simulink model "flyWheel"  (R2018b)
settings: Solver=ode45  StartTime=0.0  StopTime=59  RelTol=1e-3
libraries: simulink x3
settings Model: Creator=ROG  LastModifiedBy=ROG

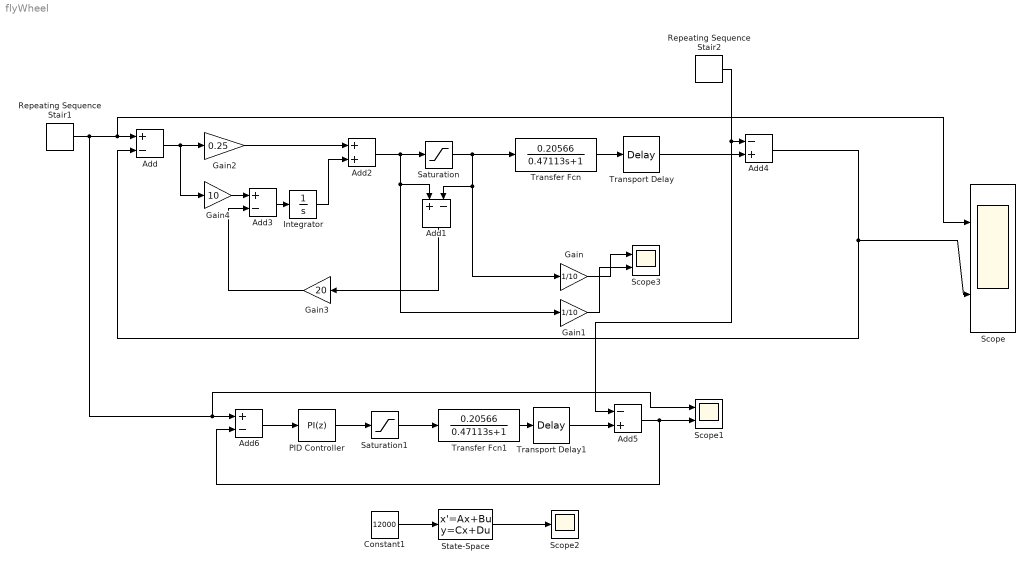
== system flyWheel ==
  Add{,1,3,6} (4 alike) : Sum  Inputs=+-
  Add2 : Sum
  Add4 : Sum  Inputs=-+
  Add5 : Sum  Inputs=-+
  Constant1 : Constant  Value=12000
  Gain : Gain  Gain=1/10
  Gain1 : Gain  Gain=1/10
  Gain2 : Gain  Gain=0.25
  Gain3 : Gain  Gain=20
  Gain4 : Gain  Gain=10
  Integrator : Integrator
  PID Controller : simulink/Continuous/PID Controller  Controller=PI  Form=Parallel  TimeDomain=Discrete-time  SampleTime=0.005  IntegratorMethod=Forward Euler  FilterMethod=Forward Euler  ControllerParametersSource=internal  P=0.25  I=10  D=0  UseFilter=on  N=100  TunerSelectOption=Transfer Function Based (PID Tuner App)  InitialConditionSource=internal  InitialConditionForIntegrator=0  InitialConditionForFilter=0  DifferentiatorICPrevScaledInput=0  ExternalReset=none  TrackingMode=off  Kt=1  LimitOutput=off  UpperSaturationLimit=inf  LowerSaturationLimit=-inf  LinearizeAsGain=on  AntiWindupMode=none  Kb=1  POutMin=[]  POutMax=[]  IOutMin=[]  IOutMax=[]  DOutMin=[]  DOutMax=[]  NOutMin=[]  NOutMax=[]  SumOutMin=[]  SumOutMax=[]  SaturationOutMin=[]  SaturationOutMax=[]  PParamMin=[]  PParamMax=[]  IParamMin=[]  IParamMax=[]  DParamMin=[]  DParamMax=[]  NParamMin=[]  NParamMax=[]  KbParamMin=[]  KbParamMax=[]  KtParamMin=[]  KtParamMax=[]  KbOutMin=[]  KbOutMax=[]  KtOutMin=[]  KtOutMax=[]  IntegratorOutMin=[]  IntegratorOutMax=[]  FilterOutMin=[]  FilterOutMax=[]  SumI1OutMin=[]  SumI1OutMax=[]  SumI2OutMin=[]  SumI2OutMax=[]  SumI3OutMin=[]  SumI3OutMax=[]  SumI4OutMin=[]  SumI4OutMax=[]  SumDOutMin=[]  SumDOutMax=[]  DifferentiatorOutMin=[]  DifferentiatorOutMax=[]  FilterDiffOutCoefMin=[]  FilterDiffOutCoefMax=[]  ReciprocalOutMin=[]  ReciprocalOutMax=[]  SumDenOutMin=[]  SumDenOutMax=[]  SumNumOutMin=[]  SumNumOutMax=[]  DivideOutMin=[]  DivideOutMax=[]  IntegratorContinuousStateAttributes=''  IntegratorStateMustResolveToSignalObject=off  IntegratorRTWStateStorageClass=Auto  FilterContinuousStateAttributes=''  FilterStateMustResolveToSignalObject=off  FilterRTWStateStorageClass=Auto  ParallelPVariant=InternalParameters  IdealPVariant=Disabled  IVariant=InternalParameters  DVariant=Disabled  IntegratorVariant=Discrete  SatVariant=Disabled  AWVariant=Passthrough  PCopyVariant=Disabled  TRVariant=Disabled  FdbkBlocksVariant=Forward  IdealPFdbkVariant=Disabled  SatFdbkVariant=Disabled  DerivativeFilterVariant=Disabled  NVariant=Disabled  NCopyVariant=Disabled_SignalSpec  FilterICVariant=Disabled  IntegratorICVariant=InternalICs  ExternalResetVariant=Disabled  TRSumVariant=Passthrough  SumFdbkVariant=Disabled  SumVariant=Sum_PI
  Repeating Sequence Stair1 : simulink/Sources/Repeating Sequence Stair  OutValues=[1800 800 2500 1800 1800].'  tsamp=10  OutMin=[]  OutMax=[]  OutDataTypeStr=double  OutputDataTypeScalingMode=double  OutDataType=fixdt(0,8)  ConRadixGroup=Best Precision: Vector-wise  OutScaling=2^-12
  Repeating Sequence Stair2 : simulink/Sources/Repeating Sequence Stair  OutValues=[0 0 0 0 600 600]  tsamp=10  OutMin=[]  OutMax=[]  OutDataTypeStr=double  OutputDataTypeScalingMode=double  OutDataType=fixdt(0,8)  ConRadixGroup=Best Precision: Vector-wise  OutScaling=2^-12
  Saturation : Saturate  UpperLimit=12000  LowerLimit=-12000
  Saturation1 : Saturate  UpperLimit=12000  LowerLimit=-12000
  Scope : Scope  NumInputPorts=2
  Scope1 : Scope  NumInputPorts=2
  Scope2 : Scope
  Scope3 : Scope  NumInputPorts=2
  State-Space : StateSpace  A=-2.1226  C=0.4365  D=0  InitialCondition=0
  Transfer Fcn : TransferFcn  Numerator=[0.20566]  Denominator=[0.47113 1]
  Transfer Fcn1 : TransferFcn  Numerator=[0.20566]  Denominator=[0.47113 1]
  Transport Delay : TransportDelay  DelayTime=0.03368
  Transport Delay1 : TransportDelay  DelayTime=0.03368
  wires:
  Transfer Fcn/1 -> Transport Delay/1
  Saturation/1 -> Gain/1, Add1/2, Transfer Fcn/1
  Add2/1 -> Gain1/1, Add1/1, Saturation/1
  Add1/1 -> Gain3/1
  Integrator/1 -> Add2/2
  Add3/1 -> Integrator/1
  Gain3/1 -> Add3/2
  Gain4/1 -> Add3/1
  Gain2/1 -> Add2/1
  Add/1 -> Gain4/1, Gain2/1
  State-Space/1 -> Scope2/1
  Constant1/1 -> State-Space/1
  Repeating Sequence Stair2/1 -> Add5/1, Add4/1
  Transport Delay/1 -> Add4/2
  Add4/1 -> Add/2, Scope/2
  Transfer Fcn1/1 -> Transport Delay1/1
  Add5/1 -> Add6/2, Scope1/2
  Repeating Sequence Stair1/1 -> Scope1/1, Add6/1, Scope/1, Add/1
  Add6/1 -> PID Controller/1
  Transport Delay1/1 -> Add5/2
  PID Controller/1 -> Saturation1/1
  Saturation1/1 -> Transfer Fcn1/1
  Gain/1 -> Scope3/1
  Gain1/1 -> Scope3/2
